simulink model "z2 (1)"  (R2017b)
settings: Solver=FixedStepDiscrete  StartTime=0.0  StopTime=0.0  RelTol=1e-3
libraries: CPOiS_SourcesSinks x6, CPOiS_DataManipulation x2
settings Model: Creator=alis  LastModifiedBy=alis

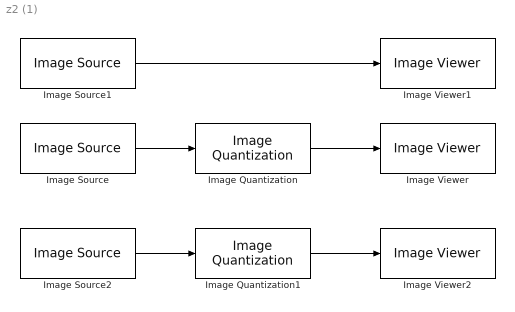
== system z2 (1) ==
  Image Quantization : CPOiS_DataManipulation/Image Quantization  LevelsNum=5
      settings: SourceProductName=CPOiS - Digital image and signal processing
  Image Quantization1 : CPOiS_DataManipulation/Image Quantization  LevelsNum=2
      settings: SourceProductName=CPOiS - Digital image and signal processing
  Image Source : CPOiS_SourcesSinks/Image Source  FileSelection=gull.png
      settings: SourceProductName=CPOiS - Digital image and signal processing
  Image Source1 : CPOiS_SourcesSinks/Image Source  FileSelection=gull.png
      settings: SourceProductName=CPOiS - Digital image and signal processing
  Image Source2 : CPOiS_SourcesSinks/Image Source  FileSelection=gull.png
      settings: SourceProductName=CPOiS - Digital image and signal processing
  Image Viewer : CPOiS_SourcesSinks/Image Viewer
      settings: SourceProductName=CPOiS - Digital image and signal processing
  Image Viewer1 : CPOiS_SourcesSinks/Image Viewer
      settings: SourceProductName=CPOiS - Digital image and signal processing
  Image Viewer2 : CPOiS_SourcesSinks/Image Viewer
      settings: SourceProductName=CPOiS - Digital image and signal processing
  wires:
  Image Source/1 -> Image Quantization/1
  Image Quantization/1 -> Image Viewer/1
  Image Source1/1 -> Image Viewer1/1
  Image Source2/1 -> Image Quantization1/1
  Image Quantization1/1 -> Image Viewer2/1
